simulink model "Task_3"  (R2020b)
settings: Solver=FixedStepDiscrete  StartTime=0.0  StopTime=10.0  RelTol=1e-3
settings Model: Creator=hp  LastModifiedBy=hp
settings OptimizationCC: DefaultParameterBehavior=Inlined  EnhancedBackFolding=on  PassReuseOutputArgsAs=Individual arguments  ZeroExternalMemoryAtStartup=off  ZeroInternalMemoryAtStartup=off  OptimizeBlockOrder=speed  DifferentSizesBufferReuse=on  OptimizationCustomize=off  EfficientTunableParamExpr=on
settings DebuggingCC: UnderspecifiedInitializationDetection=Classic  MergeDetectMultiDrivingBlocksExec=none  ParameterTunabilityLossMsg=error
settings ModelReferenceCC: PropagateSignalLabelsOutOfModel=off
settings SFSimCC: MATLABDynamicMemAlloc=off
settings RTWCC: Description=Create Visual C/C++ Solution File for Embedded Coder  SystemTargetFile=ert.tlc  GenCodeOnly=on  TemplateMakefile=RTW.MSVCBuild  GenerateReport=on  IncludeHyperlinkInReport=on  LaunchReport=on  GenerateTraceInfo=on  GenerateTraceReport=on  GenerateTraceReportSl=on  GenerateTraceReportSf=on  GenerateTraceReportEml=on  GenerateCodeReplacementReport=on
settings CodeAppCC: ForceParamTrailComments=on  IgnoreCustomStorageClasses=off  OperatorAnnotations=on  SimulinkDataObjDesc=on  SFDataObjDesc=on  InsertBlockDesc=on
settings ERTTargetCC: TargetLangStandard=C99 (ISO)  GenerateSampleERTMain=on  InlinedParameterPlacement=NonHierarchical  ERTCustomFileTemplate=example_file_process.tlc

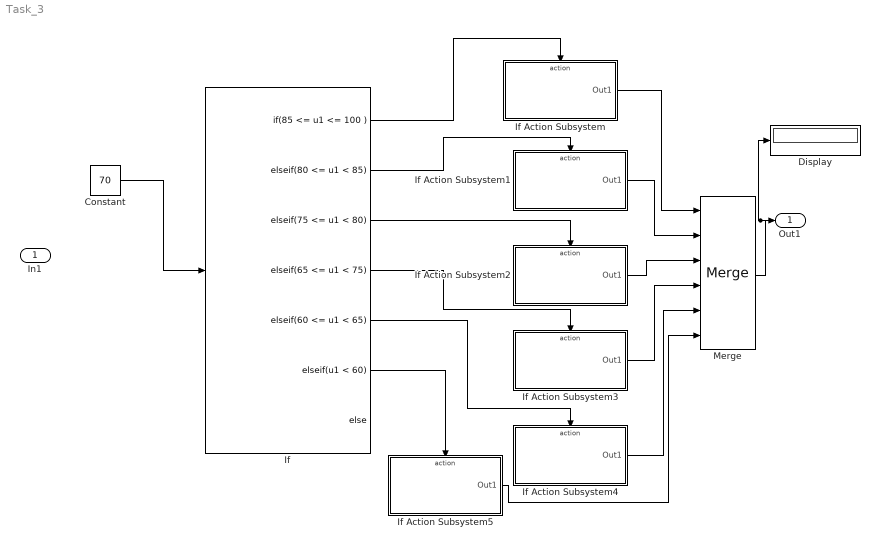
== system Task_3 ==
  In1 : Inport
  Constant : Constant  Value=70  OutDataTypeStr=uint8
  Display : Display
  If : If  IfExpression=85 <= u1 <= 100  ElseIfExpressions=80 <= u1 < 85 , 75 <= u1 < 80,65 <= u1 < 75,60 <= u1 < 65,u1 < 60
  If Action Subsystem : Subsystem  TreatAsAtomicUnit=on
  If Action Subsystem1 : Subsystem  TreatAsAtomicUnit=on
  If Action Subsystem2 : Subsystem  TreatAsAtomicUnit=on
  If Action Subsystem3 : Subsystem  TreatAsAtomicUnit=on
  If Action Subsystem4 : Subsystem  TreatAsAtomicUnit=on
  If Action Subsystem5 : Subsystem  TreatAsAtomicUnit=on
  Merge : Merge  Inputs=6
  Out1 : Outport
  wires:
  If/1 -> If Action Subsystem/Action
  If/2 -> If Action Subsystem1/Action
  If/3 -> If Action Subsystem2/Action
  If/4 -> If Action Subsystem3/Action
  If/5 -> If Action Subsystem4/Action
  If/6 -> If Action Subsystem5/Action
  If Action Subsystem/1(Out1) -> Merge/1
  If Action Subsystem1/1(Out1) -> Merge/2
  If Action Subsystem2/1(Out1) -> Merge/3
  If Action Subsystem3/1(Out1) -> Merge/4
  If Action Subsystem4/1(Out1) -> Merge/5
  If Action Subsystem5/1(Out1) -> Merge/6
  Merge/1 -> Display/1, Out1/1
  Constant/1 -> If/1

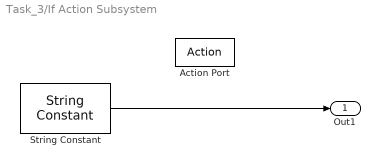
== system Task_3/If Action Subsystem ==
  Action Port : ActionPort  ActionPortLabel=if(85 <= u1 <= 100 )
  String Constant : StringConstant  String="\"Excellent\""
  Out1 : Outport
  wires:
  String Constant/1 -> Out1/1

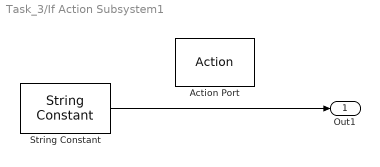
== system Task_3/If Action Subsystem1 ==
  Action Port : ActionPort  ActionPortLabel=elseif(80 <= u1 < 85 )
  String Constant : StringConstant  String="\"Very Good \""
  Out1 : Outport
  wires:
  String Constant/1 -> Out1/1

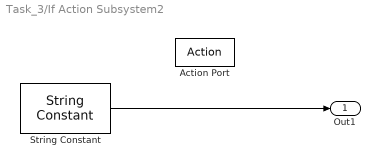
== system Task_3/If Action Subsystem2 ==
  Action Port : ActionPort  ActionPortLabel=elseif( 75 <= u1 < 80)
  String Constant : StringConstant  String="\"Good\""
  Out1 : Outport
  wires:
  String Constant/1 -> Out1/1

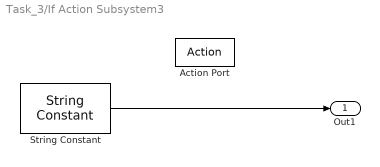
== system Task_3/If Action Subsystem3 ==
  Action Port : ActionPort  ActionPortLabel=elseif(65 <= u1 < 75)
  String Constant : StringConstant  String="\"Good\""
  Out1 : Outport
  wires:
  String Constant/1 -> Out1/1

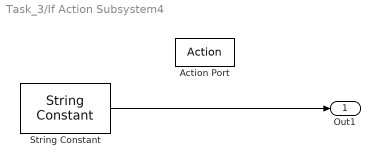
== system Task_3/If Action Subsystem4 ==
  Action Port : ActionPort  ActionPortLabel=elseif(60 <= u1 < 65)
  String Constant : StringConstant  String="\"Successed\""
  Out1 : Outport
  wires:
  String Constant/1 -> Out1/1

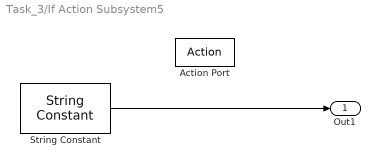
== system Task_3/If Action Subsystem5 ==
  Action Port : ActionPort  ActionPortLabel=elseif(u1 < 60)
  String Constant : StringConstant  String="\"Failed\""
  Out1 : Outport
  wires:
  String Constant/1 -> Out1/1
